simulink model "model_unutar_automobila"  (R2015b)
settings: Solver=VariableStepAuto  StartTime=0.0  StopTime=10.0  RelTol=1e-3
values from neighbouring files (symbols this model uses):
  C = 0.5    [Bode Plot.m]
undefined symbols (not defined in the file or in its folder): Imax
libraries: dspfdesign x1
settings Model: Creator=Luka  LastModifiedBy=Luka

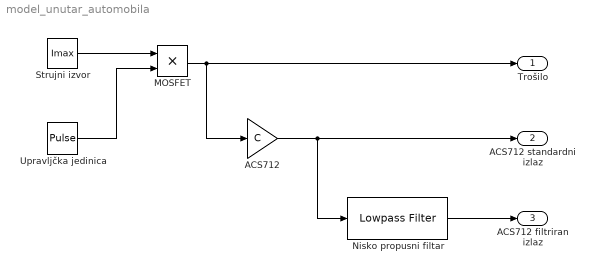
== system model_unutar_automobila ==
  ACS712 : Gain  Gain=C
  MOSFET : Product
  Nisko propusni filtar : dspfdesign/Lowpass Filter  FilterType=FIR  DesignForMinimumOrder=on  FilterOrder=50  PassbandFrequency=8e3  StopbandFrequency=12e3  PassbandRipple=0.1  StopbandAttenuation=80  InheritSampleRate=off  SampleRate=44100  roundingMode=Floor  coeffsDataTypeStr=fixdt(1,16)  SimulateUsing=Interpreted execution
  Strujni izvor : Constant  Value=Imax
  "Upravljčka jedinica " : DiscretePulseGenerator  PulseType=Time based  Period=10  PulseWidth=5
  Trošilo : Outport
  ACS712 standardni izlaz : Outport  Port=2
  ACS712 filtriran izlaz : Outport  Port=3
  wires:
  "Upravljčka jedinica "/1 -> MOSFET/2
  Strujni izvor/1 -> MOSFET/1
  MOSFET/1 -> Trošilo/1, ACS712/1
  ACS712/1 -> Nisko propusni filtar/1, ACS712 standardni izlaz/1
  Nisko propusni filtar/1 -> ACS712 filtriran izlaz/1
